simulink model "txrx_local_optim_example"  (R2023a)
settings: Solver=FixedStepDiscrete  StartTime=0.0  StopTime=200  RelTol=1e-3
undefined symbols (not defined in the file or in its folder): a, b, c
libraries: simulink x4, hdlsllib x3
settings Model: DataTypeOverride=Off  Creator=darenlee  LastModifiedBy=cchung
settings SolverCC: AlgebraicLoopSolver=TrustRegion
settings OptimizationCC: BlockReduction=off  ConditionallyExecuteInputs=off  DefaultParameterBehavior=Inlined
settings DebuggingCC: AlgebraicLoopMsg=error  SingleTaskRateTransMsg=error  UnconnectedInputMsg=warning  UnconnectedOutputMsg=warning  UnconnectedLineMsg=warning
settings HardwareCC: ProdBitPerPointer=32  ProdBitPerSizeT=32  ProdBitPerPtrDiffT=32  ProdLargestAtomicFloat=None  ProdIntDivRoundTo=Undefined  ProdEndianess=Unspecified  ProdWordSize=32  ProdHWDeviceType=ASIC/FPGA->ASIC/FPGA  TargetBitPerPointer=64  TargetBitPerSizeT=64  TargetBitPerPtrDiffT=64  TargetLongLongMode=on  TargetIntDivRoundTo=Zero  TargetEndianess=LittleEndian  TargetWordSize=64  TargetHWDeviceType=Custom Processor->MATLAB Host Computer  ProdEqTarget=off
settings ModelReferenceCC: EnableRefExpFcnMdlSchedulingChecks=on

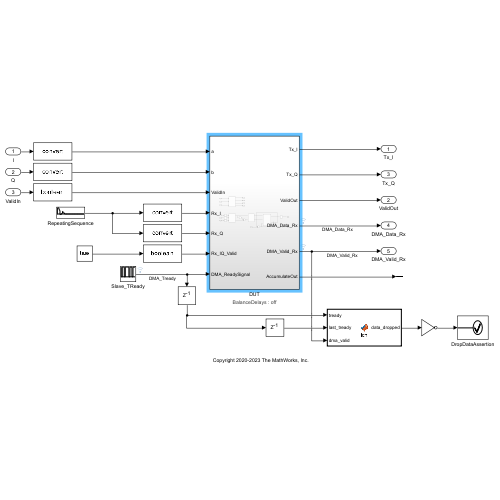
[thumbnail: Simulink's stored preview of the top-level diagram]
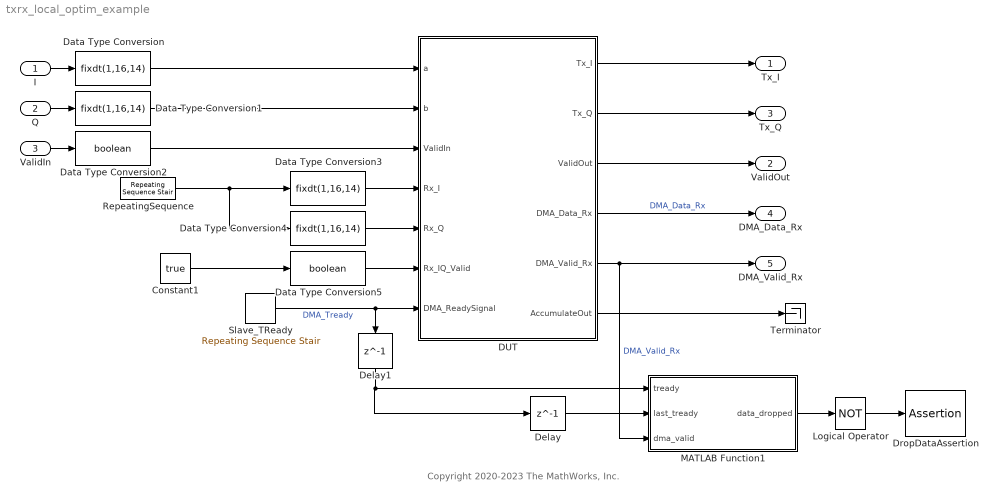
== system txrx_local_optim_example ==
  note: Copyright 2020-2023 The MathWorks, Inc.
  I : Inport
  Q : Inport  Port=2
  ValidIn : Inport  Port=3
  Constant1 : Constant  Value=true  SampleTime=1
  DUT : Subsystem
      settings: AttributesFormatString=BalanceDelays : off
  Data Type Conversion{,1,3..4} (4 alike) : DataTypeConversion  OutDataTypeStr=fixdt(1,16,14)  SaturateOnIntegerOverflow=off  RndMeth=Floor
  Data Type Conversion2 : DataTypeConversion  OutDataTypeStr=boolean  SaturateOnIntegerOverflow=off  RndMeth=Floor
  Data Type Conversion5 : DataTypeConversion  OutDataTypeStr=boolean  SaturateOnIntegerOverflow=off  RndMeth=Floor
  Delay : Delay  DelayLength=1
  Delay1 : Delay  DelayLength=1
  DropDataAssertion : Assertion
  Logical Operator : Logic  Operator=NOT  IconShape=distinctive  AllPortsSameDT=off  OutDataTypeStr=boolean
  MATLAB Function1 : MATLAB Function  TreatAsAtomicUnit=on
  RepeatingSequence : simulink/Sources/Repeating Sequence Stair  OutValues=[1.9 1.8 1.3 1.1 -0.3 -0.2 0.001 0.25 0.7 0.3 0.2 0.001 zeros(1,30)]  tsamp=-1  OutMin=[]  OutMax=[]  OutDataTypeStr=double  OutputDataTypeScalingMode=double  OutDataType=fixdt(0,8)  ConRadixGroup=Best Precision: Vector-wise  OutScaling=2^-12
  Slave_TReady : simulink/Sources/Repeating Sequence Stair  OutValues=[0 1 1 0 1 1 1 0 1 1 0 1 1 ].'  tsamp=-1  OutMin=[]  OutMax=[]  OutDataTypeStr=fixdt('boolean')  OutputDataTypeScalingMode=Specify via dialog  OutDataType=fixdt('boolean')  ConRadixGroup=Best Precision: Vector-wise  OutScaling=[]
  Terminator : Terminator
  Tx_I : Outport
  ValidOut : Outport  Port=2
  Tx_Q : Outport  Port=3
  DMA_Data_Rx : Outport  Port=4
  DMA_Valid_Rx : Outport  Port=5
  wires:
  I/1 -> Data Type Conversion/1
  Q/1 -> Data Type Conversion1/1
  ValidIn/1 -> Data Type Conversion2/1
  DUT/1(Tx_I) -> Tx_I/1
  DUT/3(ValidOut) -> ValidOut/1
  Data Type Conversion/1 -> DUT/1(a)
  Data Type Conversion1/1 -> DUT/2(b)
  DUT/2(Tx_Q) -> Tx_Q/1
  Data Type Conversion2/1 -> DUT/3(ValidIn)
  Constant1/1 -> Data Type Conversion5/1
  RepeatingSequence/1 -> Data Type Conversion4/1, Data Type Conversion3/1
  Data Type Conversion3/1 -> DUT/4(Rx_I)
  Data Type Conversion4/1 -> DUT/5(Rx_Q)
  Data Type Conversion5/1 -> DUT/6(Rx_IQ_Valid)
  Slave_TReady/1 -> Delay1/1, DUT/7(DMA_ReadySignal)  "DMA_Tready"
  DUT/4(DMA_Data_Rx) -> DMA_Data_Rx/1  "DMA_Data_Rx"
  DUT/5(DMA_Valid_Rx) -> MATLAB Function1/3(dma_valid), DMA_Valid_Rx/1  "DMA_Valid_Rx"
  Delay/1 -> MATLAB Function1/2(last_tready)
  Delay1/1 -> MATLAB Function1/1(tready), Delay/1
  MATLAB Function1/1(data_dropped) -> Logical Operator/1
  Logical Operator/1 -> DropDataAssertion/1
  DUT/6(AccumulateOut) -> Terminator/1

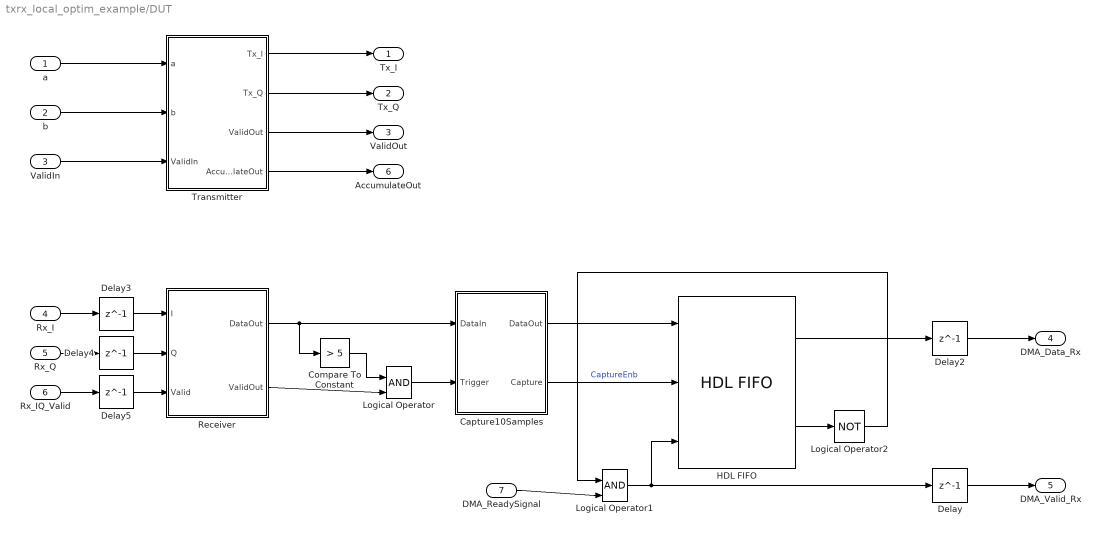
== system txrx_local_optim_example/DUT ==
  a : Inport
  b : Inport  Port=2
  ValidIn : Inport  Port=3
  Rx_I : Inport  Port=4
  Rx_Q : Inport  Port=5
  Rx_IQ_Valid : Inport  Port=6
  DMA_ReadySignal : Inport  Port=7
  Capture10Samples : Subsystem
  Compare To Constant : simulink/Logic and Bit Operations/Compare To Constant  relop=>  const=5  OutDataTypeStr=boolean
  Delay{,2..5} (5 alike) : Delay  DelayLength=1
  HDL FIFO : hdlsllib/HDL RAMs/HDL FIFO  fifo_size=1024  mode=FWFT  ratio=1  push_msg=Warning  pop_msg=Warning  show_empty=on  show_full=off  show_num=off  LabelModeActiveChoice_Mode=FWFT  rst_port=off
  Logical Operator : Logic  IconShape=distinctive  AllPortsSameDT=off  OutDataTypeStr=boolean
  Logical Operator1 : Logic  IconShape=distinctive  AllPortsSameDT=off  OutDataTypeStr=boolean
  Logical Operator2 : Logic  Operator=NOT  IconShape=distinctive  AllPortsSameDT=off  OutDataTypeStr=boolean
  Receiver : Subsystem
      settings: AttributesFormatString=|
      | AdaptivePipelining : on
      | BalanceDelays : on
  Transmitter : Subsystem
      settings: AttributesFormatString=BalanceDelays : on
  Tx_I : Outport
  Tx_Q : Outport  Port=2
  ValidOut : Outport  Port=3
  DMA_Data_Rx : Outport  Port=4
  DMA_Valid_Rx : Outport  Port=5
  AccumulateOut : Outport  Port=6
  wires:
  a/1 -> Transmitter/1(a)
  b/1 -> Transmitter/2(b)
  ValidIn/1 -> Transmitter/3(ValidIn)
  Rx_I/1 -> Delay3/1
  Rx_Q/1 -> Delay4/1
  Rx_IQ_Valid/1 -> Delay5/1
  Receiver/1(DataOut) -> Capture10Samples/1(DataIn), Compare To Constant/1
  Receiver/2(ValidOut) -> Logical Operator/2
  Compare To Constant/1 -> Logical Operator/1
  Logical Operator/1 -> Capture10Samples/2(Trigger)
  HDL FIFO/2 -> Logical Operator2/1
  Logical Operator2/1 -> Logical Operator1/1
  Logical Operator1/1 -> HDL FIFO/3, Delay/1
  DMA_ReadySignal/1 -> Logical Operator1/2
  HDL FIFO/1 -> Delay2/1
  Capture10Samples/2(Capture) -> HDL FIFO/2  "CaptureEnb"
  Capture10Samples/1(DataOut) -> HDL FIFO/1
  Delay/1 -> DMA_Valid_Rx/1
  Delay2/1 -> DMA_Data_Rx/1
  Delay3/1 -> Receiver/1(I)
  Delay4/1 -> Receiver/2(Q)
  Delay5/1 -> Receiver/3(Valid)
  Transmitter/1(Tx_I) -> Tx_I/1
  Transmitter/2(Tx_Q) -> Tx_Q/1
  Transmitter/3(ValidOut) -> ValidOut/1
  Transmitter/4(AccumulateOut) -> AccumulateOut/1

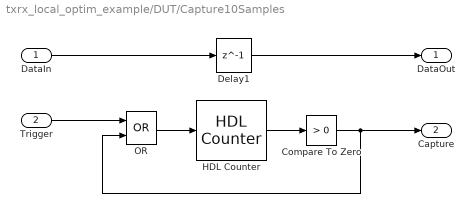
== system txrx_local_optim_example/DUT/Capture10Samples ==
  DataIn : Inport
  Trigger : Inport  Port=2
  Compare To Zero : simulink/Logic and Bit Operations/Compare To Zero  relop=>  OutDataTypeStr=boolean
  Delay1 : Delay  DelayLength=1
  HDL Counter : hdlsllib/Sources/HDL Counter  CountType=Count limited  CountInit=0  CountStep=1  CountMax=10  CountFromType=Initial value  CountFrom=0  CountResetPort=off  CountLoadPort=off  CountEnbPort=on  CountDirPort=off  CountHitOutputPort=off  CountDataType=Unsigned  CountWordLen=8  CountFracLen=0  CountSampTime=1
  OR : Logic  Operator=OR  AllPortsSameDT=off  OutDataTypeStr=boolean
  DataOut : Outport
  Capture : Outport  Port=2
  wires:
  OR/1 -> HDL Counter/1
  HDL Counter/1 -> Compare To Zero/1
  Trigger/1 -> OR/1
  Compare To Zero/1 -> Capture/1, OR/2
  DataIn/1 -> Delay1/1
  Delay1/1 -> DataOut/1

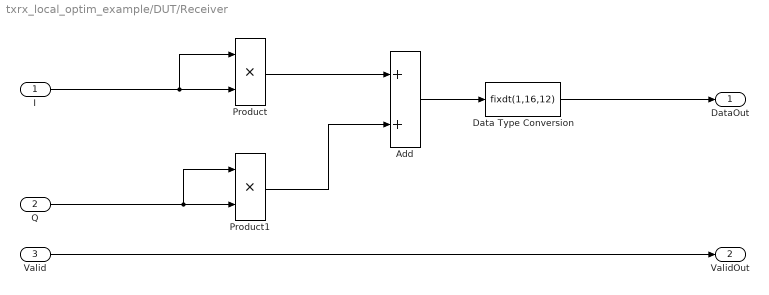
== system txrx_local_optim_example/DUT/Receiver ==
  I : Inport
  Q : Inport  Port=2
  Valid : Inport  Port=3
  Add : Sum
  Data Type Conversion : DataTypeConversion  OutDataTypeStr=fixdt(1,16,12)  SaturateOnIntegerOverflow=off  RndMeth=Floor
  Product : Product
  Product1 : Product
  DataOut : Outport
  ValidOut : Outport  Port=2
  wires:
  I/1 -> Product/1, Product/2
  Data Type Conversion/1 -> DataOut/1
  Q/1 -> Product1/1, Product1/2
  Valid/1 -> ValidOut/1
  Add/1 -> Data Type Conversion/1
  Product/1 -> Add/1
  Product1/1 -> Add/2

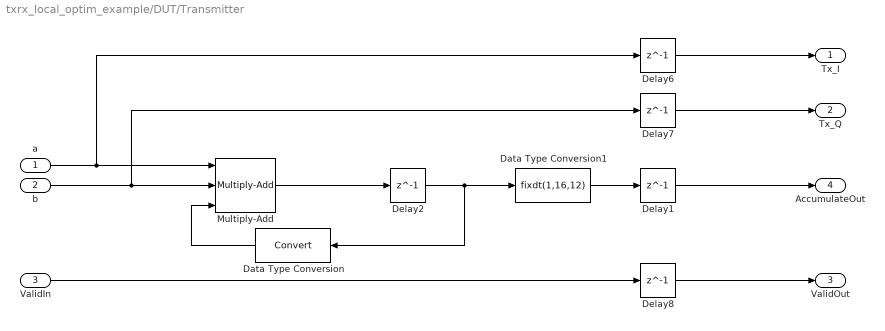
== system txrx_local_optim_example/DUT/Transmitter ==
  a : Inport
  b : Inport  Port=2
  ValidIn : Inport  Port=3
  Data Type Conversion : DataTypeConversion  SaturateOnIntegerOverflow=off  RndMeth=Floor
  Data Type Conversion1 : DataTypeConversion  OutDataTypeStr=fixdt(1,16,12)  SaturateOnIntegerOverflow=off  RndMeth=Floor
  Delay{1..2,6..8} (5 alike) : Delay  DelayLength=1
  Multiply-Add : hdlsllib/HDL Operations/Multiply-Add  Function=c+(a.*b)  datatype=Inherit: Inherit via internal rule  DoSatur=off  FMA=off
  Tx_I : Outport
  Tx_Q : Outport  Port=2
  ValidOut : Outport  Port=3
  AccumulateOut : Outport  Port=4
  wires:
  a/1 -> Delay6/1, Multiply-Add/1
  Multiply-Add/1 -> Delay2/1
  Delay1/1 -> AccumulateOut/1
  Data Type Conversion1/1 -> Delay1/1
  b/1 -> Delay7/1, Multiply-Add/2
  Delay2/1 -> Data Type Conversion1/1, Data Type Conversion/1
  Data Type Conversion/1 -> Multiply-Add/3
  ValidIn/1 -> Delay8/1
  Delay8/1 -> ValidOut/1
  Delay6/1 -> Tx_I/1
  Delay7/1 -> Tx_Q/1

== matlab function txrx_local_optim_example/MATLAB Function1 ==
  settings: fimath=hdlfimath
  data: tready input; data_dropped output; last_tready input; dma_valid input
function data_dropped = fcn(tready, last_tready, dma_valid)
% persistent last_state
data_dropped = false;
if tready == false && last_tready == true
    if dma_valid
        data_dropped = true;
  
    end
end
